simulink model "lab3_model"  (R2015a)
settings: Solver=ode4  SolverMode=SingleTasking  StartTime=0.0  StopTime=10.0  FixedStep=1e-2  RelTol=1e-3
values from neighbouring files (symbols this model uses):
  A = [ -2  0 ... (first row only)    [script.m]    (also in script1.m = 1; script2.m = Ap; script3.m = [0 1;-5 -8])
  B = [ -1 ... (first row only)    [script.m]    (also in script2.m = Bp; script3.m = [0;1])
  C = [ 1.5 0.2 ]    [script.m]    (also in script2.m = eye(2); script3.m = eye(2))
  D = [0;0]    [script2.m]
  WPC = 1    [script2.m]    (also in script3.m = 0)
settings Model: Creator=bb  LastModifiedBy=bb
settings DataIOCC: LimitDataPoints=off

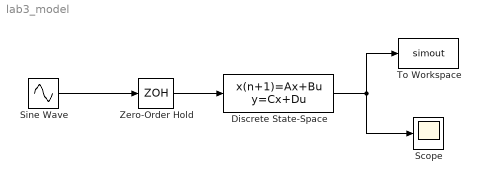
== system lab3_model ==
  Discrete State-Space : DiscreteStateSpace  A=A  B=B  C=C  D=D  X0=WPC
  Scope : Scope
  Sine Wave : Sin  SampleTime=0
  To Workspace : ToWorkspace  VariableName=simout  SaveFormat=Timeseries  SampleTime=-1
  Zero-Order Hold : ZeroOrderHold
  wires:
  Zero-Order Hold/1 -> Discrete State-Space/1
  Discrete State-Space/1 -> To Workspace/1, Scope/1
  Sine Wave/1 -> Zero-Order Hold/1
